simulink subsystem "into_wave"  (R2025b)
settings: Solver=VariableStepAuto  StartTime=0.0  StopTime=10.0  RelTol=1e-3
settings Model: Creator=sanborkl  LastModifiedBy=jdcjdb

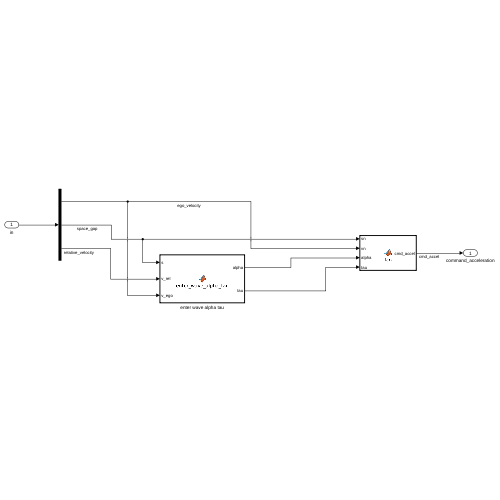
[thumbnail: Simulink's stored preview of the top-level diagram]
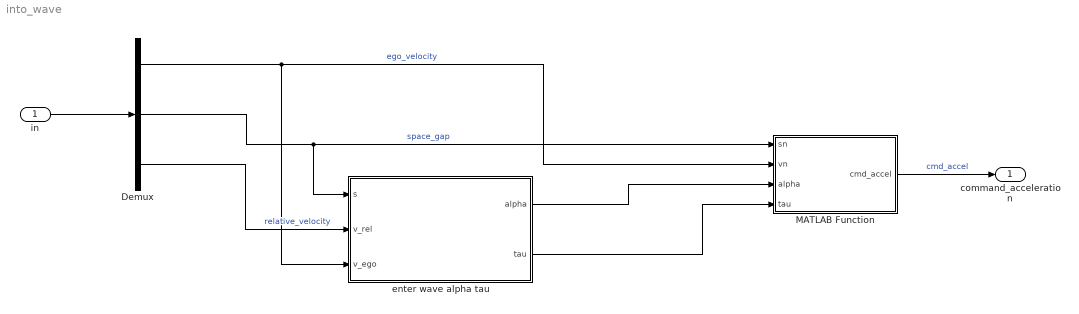
== system into_wave ==
  in : Inport
  Demux : Demux  Outputs=3
  MATLAB Function : MATLAB Function  TreatAsAtomicUnit=on
  enter wave alpha tau : MATLAB Function  TreatAsAtomicUnit=on
  command_acceleration : Outport
  wires:
  Demux/2 -> enter wave alpha tau/1(s), MATLAB Function/1(sn)  "space_gap"
  Demux/1 -> enter wave alpha tau/3(v_ego), MATLAB Function/2(vn)  "ego_velocity"
  Demux/3 -> enter wave alpha tau/2(v_rel)  "relative_velocity"
  in/1 -> Demux/1
  MATLAB Function/1(cmd_accel) -> command_acceleration/1  "cmd_accel"
  enter wave alpha tau/1(alpha) -> MATLAB Function/3(alpha)
  enter wave alpha tau/2(tau) -> MATLAB Function/4(tau)

== matlab function into_wave/enter wave alpha tau ==
  data: s input; alpha output; v_rel input; v_ego input; tau output
function [alpha, tau] = enter_wave_alpha_tau(s, v_rel, v_ego)
%#codegen
% ENTER-WAVE: Increase tau and reduce alpha when closing in or the gap is short.
% Inputs:
%   s      [m]   space gap
%   v_rel  [m/s] v_lead - v_ego  (negative when closing)
%   v_ego  [m/s] ego speed
% Outputs:
%   alpha  [-]   weight for spacing term (0..1)
%   tau    [s]   time gap

% ===== Tunables =====
s0         = 2.0;    % [m] standstill distance
tau_base   = 1.6;    % [s] base headway in Enter
tau_min    = 0.9;    % [s]
tau_max    = 2.4;    % [s]

alpha_base = 0.65;   % [-]
alpha_min  = 0.25;   % [-]
alpha_max  = 0.95;   % [-]

% Reactivity (how strongly to adapt):
k_tau_rel  = 0.10;   % [s^2/m]  tau += k * (-v_rel)+
k_tau_gap  = 0.04;   % [s/m]    tau += k * (s_des0 - s)+
k_a_rel    = 0.20;   % [-/(m/s)] alpha -= k * (-v_rel)+
k_a_gap    = 0.04;   % [-/m]     alpha -= k * (s_des0 - s)+

% Smoothing
Ts         = 0.01;   % [s] sample time
T_alpha    = 0.25;   % [s] LPF time-constant for alpha
T_tau      = 0.25;   % [s] LPF time-constant for tau
% =====================

% Desired gap with base tau (reference for "short-gap")
s_des0   = s0 + tau_base * v_ego;
closing  = max(-v_rel, 0.0);        % m/s (only when closing)
shortgap = max( s_des0 - s, 0.0 );  % m  (only when too close)

% Raw (unfiltered) targets
tau_tgt   = clamp(tau_base   + k_tau_rel*closing + k_tau_gap*shortgap, tau_min,  tau_max);
alpha_tgt = clamp(alpha_base - k_a_rel*closing   - k_a_gap*shortgap,   alpha_min, alpha_max);

% First-order smoothing on outputs
persistent alpha_prev tau_prev
if isempty(alpha_prev); alpha_prev = alpha_tgt; end
if isempty(tau_prev);   tau_prev   = tau_tgt;   end

b_a = (T_alpha > 1e-6) * (Ts/(T_alpha+Ts)) + (T_alpha <= 1e-6) * 1.0;
b_t = (T_tau   > 1e-6) * (Ts/(T_tau  +Ts)) + (T_tau   <= 1e-6) * 1.0;

alpha = alpha_prev + b_a * (alpha_tgt - alpha_prev);
tau   = tau_prev   + b_t * (tau_tgt   - tau_prev);

alpha_prev = alpha;
tau_prev   = tau;

% --- helper ---
function y = clamp(x, lo, hi)
%#codegen
y = min(max(x, lo), hi);
end
end

== matlab function into_wave/MATLAB Function ==
  data: sn input; cmd_accel output; vn input; alpha input; tau input
function cmd_accel = fcn(sn, vn, alpha, tau)

cmd_accel = alpha * (sn - tau * vn);
